simulink model "quadcopter"  (R2024a)
settings: Solver=ode45  StartTime=0.0  StopTime=100  FixedStep=0.0001  RelTol=1e-3
libraries: slpidlib x9
(part 1 of 2)
settings Model: Creator=ADMIN  LastModifiedBy=ADMIN

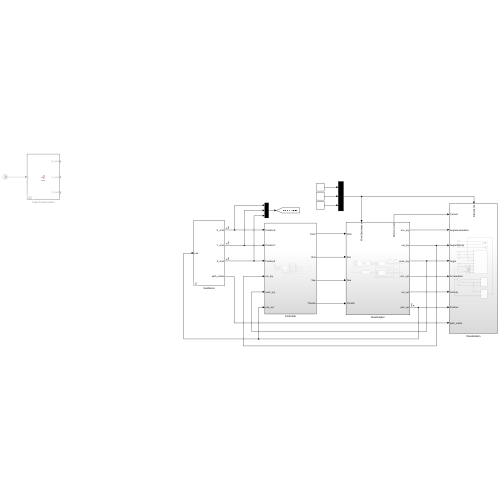
[thumbnail: Simulink's stored preview of the top-level diagram]
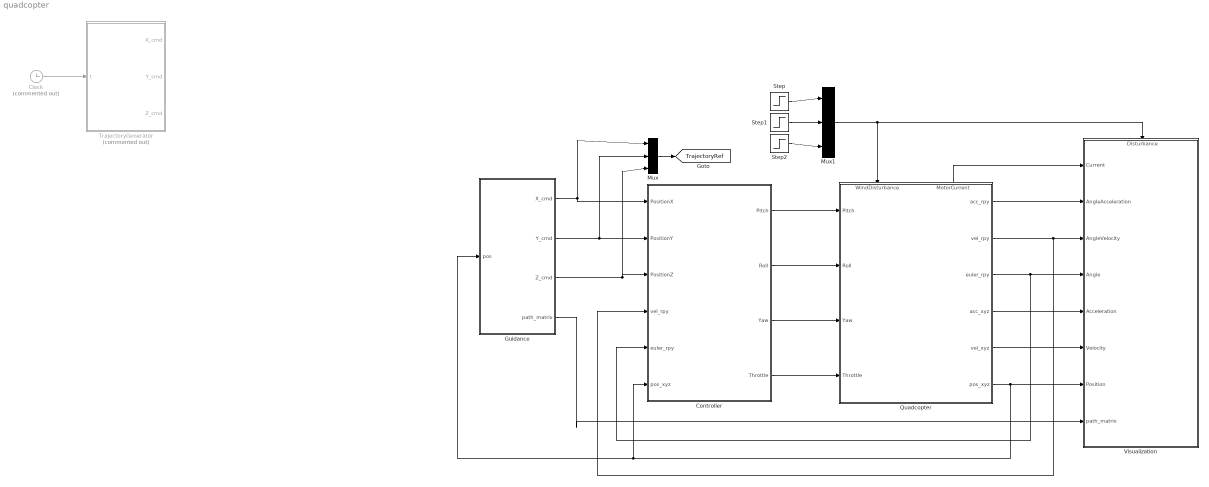
== system quadcopter ==
  Clock : Clock  Commented=on
  Controller : Subsystem
  Guidance : Subsystem  mask{trajectory_type=1}
      mask prompts: trajectory_type "helix: 1, figure-8: 2"
  Mux : Mux  Inputs=3
  Mux1 : Mux  Inputs=3
  Quadcopter : Subsystem
      settings: PortSchema="{\"entries\":[{\"content\":{\"sides\":[{\"content\":{\"connectorIds\":[\"In1\",\"In2\",\"In3\",\"In4\"]},\"type\":\"ConnectorPlacement.EquallySpacedRectSide\",\"uuid\":\"72979afb-3a13-47a6-b2df-41b5587480e1\"},{\"content\":{\"connectorIds\":[\"Out1\",\"Out2\",\"Out3\",\"Out4\",\"Out5\",\"Out6\"],\"side\":\"RIGHT\"},\"type\":\"ConnectorPlacement.EquallySpacedRectSide\",\"uuid\":\"ea12cd5a-a884-45c1-8d68-b4383d709346\"},{\"content\":{\"connectorIds\":[\"In5\",\"Out7\"],\"side\":\"TOP\"},\"type\":\"ConnectorPlacement.EquallySpacedRectSide\",\"uuid\":\"9fa1b2a5-ed05-4359-b2a5-dd09b0942958\"}]},\"type\":\"ConnectorPlacement.EquallySpacedConnector\",\"uuid\":\"94bc8a31-e0f4-4496-86b6-9264019e9c52\"}],\"packageUris\":[\"http://schema.mathworks.com/mf0/Connector/R2020b\"],\"version\":\"1.0\"}"
  Step : Step  Time=10  After=4  SampleTime=0
  Step1 : Step  Time=40  After=0  SampleTime=0
  Step2 : Step  Time=60  After=0  SampleTime=0
  TrajectoryGenerator : MATLAB Function  Commented=on  TreatAsAtomicUnit=on
  Visualization : Subsystem
      settings: PortSchema="{\"entries\":[{\"content\":{\"sides\":[{\"content\":{\"connectorIds\":[\"In1\",\"In2\",\"In3\",\"In4\",\"In5\",\"In6\",\"In7\",\"In8\"]},\"type\":\"ConnectorPlacement.EquallySpacedRectSide\",\"uuid\":\"3cb0b979-0d5f-4f09-adcd-90aa91650358\"},{\"content\":{\"side\":\"RIGHT\"},\"type\":\"ConnectorPlacement.EquallySpacedRectSide\",\"uuid\":\"d4f03e78-8acd-4062-a16e-5eca778df7bc\"},{\"content\":{\"connectorIds\":[\"In9\"],\"side\":\"TOP\"},\"type\":\"ConnectorPlacement.EquallySpacedRectSide\",\"uuid\":\"69a143a0-3c25-4fd4-9005-042b32bb0dbc\"}]},\"type\":\"ConnectorPlacement.EquallySpacedConnector\",\"uuid\":\"bd282390-c963-4ab6-a9ae-6b9e051d8e4c\"}],\"packageUris\":[\"http://schema.mathworks.com/mf0/Connector/R2020b\"],\"version\":\"1.0\"}"
  tag scope: TrajectoryRef=global
  wires:
  Quadcopter/6(pos_xyz) -> Guidance/1(pos), Controller/6(pos_xyz), Visualization/7(Position)
  Quadcopter/2(vel_rpy) -> Controller/4(vel_rpy), Visualization/3(AngleVelocity)
  Quadcopter/3(euler_rpy) -> Controller/5(euler_rpy), Visualization/4(Angle)
  Controller/1(Pitch) -> Quadcopter/1(Pitch)
  Controller/2(Roll) -> Quadcopter/2(Roll)
  Controller/3(Yaw) -> Quadcopter/3(Yaw)
  Controller/4(Throttle) -> Quadcopter/4(Throttle)
  Mux/1 -> [TrajectoryRef]
  Clock/1 -> TrajectoryGenerator/1(t)
  Guidance/3(Z_cmd) -> Controller/3(PositionZ), Mux/3
  Guidance/2(Y_cmd) -> Controller/2(PositionY), Mux/2
  Quadcopter/7(MotorCurrent) -> Visualization/1(Current)
  Quadcopter/1(acc_rpy) -> Visualization/2(AngleAcceleration)
  Guidance/4(path_matrix) -> Visualization/8(path_matrix)
  Quadcopter/4(acc_xyz) -> Visualization/5(Acceleration)
  Quadcopter/5(vel_xyz) -> Visualization/6(Velocity)
  Guidance/1(X_cmd) -> Mux/1, Controller/1(PositionX)
  Step/1 -> Mux1/1
  Step1/1 -> Mux1/2
  Step2/1 -> Mux1/3
  Mux1/1 -> Quadcopter/5(WindDisturbance), Visualization/9(Disturbance)

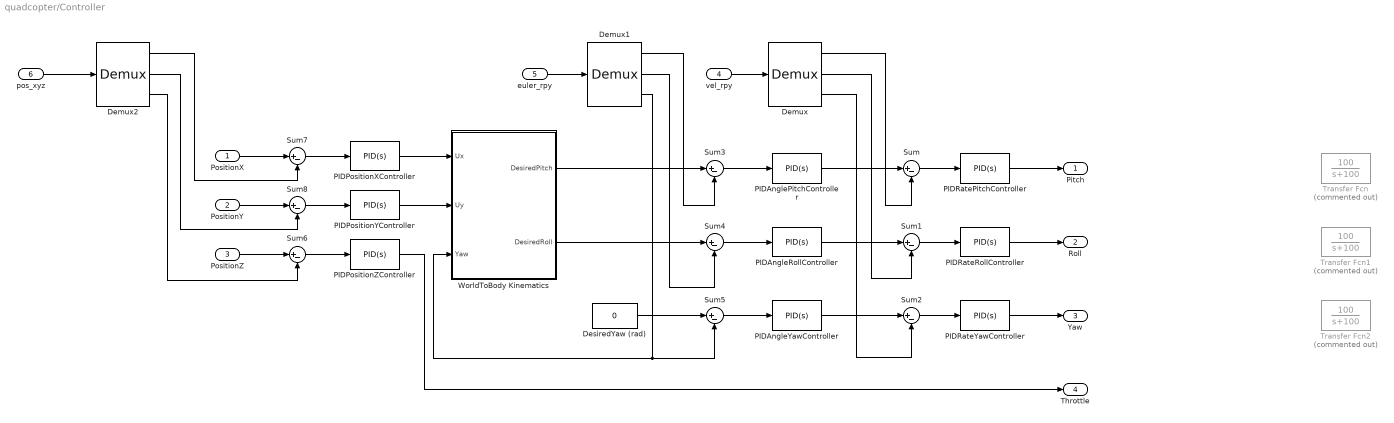
== system quadcopter/Controller ==
  PositionX : Inport
  PositionY : Inport  Port=2
  PositionZ : Inport  Port=3
  vel_rpy : Inport  Port=4
  euler_rpy : Inport  Port=5
  pos_xyz : Inport  Port=6
  Demux : Demux  Outputs=3
  Demux1 : Demux  Outputs=3
  Demux2 : Demux  Outputs=3
  DesiredYaw (rad) : Constant  Value=0
  PIDAnglePitchController : slpidlib/PID Controller  Controller=PID  Form=Parallel  TimeDomain=Continuous-time  UseExternalTs=off  SampleTime=-1  IntegratorMethod=Forward Euler  FilterMethod=Forward Euler  ControllerParametersSource=internal  P=10  I=5  UseKiTs=off  D=0  UseExternalDerivativeSource=off  N=100  UseFilter=on  TunerSelectOption=Transfer Function Based (PID Tuner App)  InitialConditionSource=internal  InitialConditionForIntegrator=0  InitialConditionForFilter=0  DifferentiatorICPrevScaledInput=0  ExternalReset=none  TrackingMode=off  Kt=1  LimitOutput=on  SatLimitsSource=internal  UpperSaturationLimit=50  LowerSaturationLimit=-50  LinearizeAsGain=on  AntiWindupMode=clamping  Kb=1  LimitIntegrator=off  UpperIntegratorSaturationLimit=inf  LowerIntegratorSaturationLimit=-inf  POutMin=[]  POutMax=[]  IOutMin=[]  IOutMax=[]  DOutMin=[]  DOutMax=[]  NOutMin=[]  NOutMax=[]  SumOutMin=[]  SumOutMax=[]  SaturationOutMin=[]  SaturationOutMax=[]  PParamMin=[]  PParamMax=[]  IParamMin=[]  IParamMax=[]  DParamMin=[]  DParamMax=[]  NParamMin=[]  NParamMax=[]  KbParamMin=[]  KbParamMax=[]  KtParamMin=[]  KtParamMax=[]  KbOutMin=[]  KbOutMax=[]  KtOutMin=[]  KtOutMax=[]  IntegratorOutMin=[]  IntegratorOutMax=[]  FilterOutMin=[]  FilterOutMax=[]  SumI1OutMin=[]  SumI1OutMax=[]  SumI2OutMin=[]  SumI2OutMax=[]  SumI3OutMin=[]  SumI3OutMax=[]  SumI4OutMin=[]  SumI4OutMax=[]  SumDOutMin=[]  SumDOutMax=[]  DifferentiatorOutMin=[]  DifferentiatorOutMax=[]  FilterDiffOutCoefMin=[]  FilterDiffOutCoefMax=[]  ReciprocalOutMin=[]  ReciprocalOutMax=[]  SumDenOutMin=[]  SumDenOutMax=[]  SumNumOutMin=[]  SumNumOutMax=[]  DivideOutMin=[]  DivideOutMax=[]  UdiffTsProdOutMin=[]  UdiffTsProdOutMax=[]  NTsProdOutMin=[]  NTsProdOutMax=[]  UintegralTsProdOutMin=[]  UintegralTsProdOutMax=[]  UngainTsProdOutMin=[]  UngainTsProdOutMax=[]  ClampingZeroOutDataTypeStr=Inherit: Inherit via back propagation  ClampingZeroOutMin=[]  ClampingZeroOutMax=[]  FilterDenConstantOutDataTypeStr=Inherit: Inherit via back propagation  FilterDenConstantOutMin=[]  FilterDenConstantOutMax=[]  PCopyOutDataTypeStr=Inherit: Inherit via back propagation  PCopyOutMin=[]  PCopyOutMax=[]  NCopyOutDataTypeStr=Inherit: Inherit via back propagation  NCopyOutMin=[]  NCopyOutMax=[]  IntegratorContinuousStateAttributes=''  IntegratorStateMustResolveToSignalObject=off  IntegratorRTWStateStorageClass=Auto  FilterContinuousStateAttributes=''  FilterStateMustResolveToSignalObject=off  FilterRTWStateStorageClass=Auto  ParallelPVariant=InternalParameters  IdealPVariant=Disabled  IVariant=InternalParameters  DVariant=InternalParameters  IntegratorVariant=Continuous  SatVariant=Enabled  AWVariant=ContClampingParallel  PCopyVariant=Disabled  TRVariant=Disabled  FdbkBlocksVariant=Forward  IdealPFdbkVariant=Disabled  SatFdbkVariant=Disabled  DerivativeFilterVariant=ContFilter  NVariant=InternalParameters  NCopyVariant=Disabled  FilterICVariant=InternalICsFilter  IntegratorICVariant=InternalICs  ExternalResetVariant=Disabled  TRSumVariant=Passthrough  SumFdbkVariant=Disabled  SumVariant=Sum_PID  TsampFilterVariant=InternalTs  TsampNgainVariant=Passthrough  TsampIntegralVariant=Disabled_SignalSpec  ExternalSaturationOutDataTypeStr=Inherit: Same as second input  DerivativeSourceVariant=ErrorSignal
  PIDAngleRollController : slpidlib/PID Controller  Controller=PID  Form=Parallel  TimeDomain=Continuous-time  UseExternalTs=off  SampleTime=-1  IntegratorMethod=Forward Euler  FilterMethod=Forward Euler  ControllerParametersSource=internal  P=10  I=5  UseKiTs=off  D=0  UseExternalDerivativeSource=off  N=100  UseFilter=on  TunerSelectOption=Transfer Function Based (PID Tuner App)  InitialConditionSource=internal  InitialConditionForIntegrator=0  InitialConditionForFilter=0  DifferentiatorICPrevScaledInput=0  ExternalReset=none  TrackingMode=off  Kt=1  LimitOutput=on  SatLimitsSource=internal  UpperSaturationLimit=50  LowerSaturationLimit=-50  LinearizeAsGain=on  AntiWindupMode=clamping  Kb=1  LimitIntegrator=off  UpperIntegratorSaturationLimit=inf  LowerIntegratorSaturationLimit=-inf  POutMin=[]  POutMax=[]  IOutMin=[]  IOutMax=[]  DOutMin=[]  DOutMax=[]  NOutMin=[]  NOutMax=[]  SumOutMin=[]  SumOutMax=[]  SaturationOutMin=[]  SaturationOutMax=[]  PParamMin=[]  PParamMax=[]  IParamMin=[]  IParamMax=[]  DParamMin=[]  DParamMax=[]  NParamMin=[]  NParamMax=[]  KbParamMin=[]  KbParamMax=[]  KtParamMin=[]  KtParamMax=[]  KbOutMin=[]  KbOutMax=[]  KtOutMin=[]  KtOutMax=[]  IntegratorOutMin=[]  IntegratorOutMax=[]  FilterOutMin=[]  FilterOutMax=[]  SumI1OutMin=[]  SumI1OutMax=[]  SumI2OutMin=[]  SumI2OutMax=[]  SumI3OutMin=[]  SumI3OutMax=[]  SumI4OutMin=[]  SumI4OutMax=[]  SumDOutMin=[]  SumDOutMax=[]  DifferentiatorOutMin=[]  DifferentiatorOutMax=[]  FilterDiffOutCoefMin=[]  FilterDiffOutCoefMax=[]  ReciprocalOutMin=[]  ReciprocalOutMax=[]  SumDenOutMin=[]  SumDenOutMax=[]  SumNumOutMin=[]  SumNumOutMax=[]  DivideOutMin=[]  DivideOutMax=[]  UdiffTsProdOutMin=[]  UdiffTsProdOutMax=[]  NTsProdOutMin=[]  NTsProdOutMax=[]  UintegralTsProdOutMin=[]  UintegralTsProdOutMax=[]  UngainTsProdOutMin=[]  UngainTsProdOutMax=[]  ClampingZeroOutDataTypeStr=Inherit: Inherit via back propagation  ClampingZeroOutMin=[]  ClampingZeroOutMax=[]  FilterDenConstantOutDataTypeStr=Inherit: Inherit via back propagation  FilterDenConstantOutMin=[]  FilterDenConstantOutMax=[]  PCopyOutDataTypeStr=Inherit: Inherit via back propagation  PCopyOutMin=[]  PCopyOutMax=[]  NCopyOutDataTypeStr=Inherit: Inherit via back propagation  NCopyOutMin=[]  NCopyOutMax=[]  IntegratorContinuousStateAttributes=''  IntegratorStateMustResolveToSignalObject=off  IntegratorRTWStateStorageClass=Auto  FilterContinuousStateAttributes=''  FilterStateMustResolveToSignalObject=off  FilterRTWStateStorageClass=Auto  ParallelPVariant=InternalParameters  IdealPVariant=Disabled  IVariant=InternalParameters  DVariant=InternalParameters  IntegratorVariant=Continuous  SatVariant=Enabled  AWVariant=ContClampingParallel  PCopyVariant=Disabled  TRVariant=Disabled  FdbkBlocksVariant=Forward  IdealPFdbkVariant=Disabled  SatFdbkVariant=Disabled  DerivativeFilterVariant=ContFilter  NVariant=InternalParameters  NCopyVariant=Disabled  FilterICVariant=InternalICsFilter  IntegratorICVariant=InternalICs  ExternalResetVariant=Disabled  TRSumVariant=Passthrough  SumFdbkVariant=Disabled  SumVariant=Sum_PID  TsampFilterVariant=InternalTs  TsampNgainVariant=Passthrough  TsampIntegralVariant=Disabled_SignalSpec  ExternalSaturationOutDataTypeStr=Inherit: Same as second input  DerivativeSourceVariant=ErrorSignal
  PIDAngleYawController : slpidlib/PID Controller  Controller=PID  Form=Parallel  TimeDomain=Continuous-time  UseExternalTs=off  SampleTime=-1  IntegratorMethod=Forward Euler  FilterMethod=Forward Euler  ControllerParametersSource=internal  P=10  I=0.5  UseKiTs=off  D=0  UseExternalDerivativeSource=off  N=100  UseFilter=on  TunerSelectOption=Transfer Function Based (PID Tuner App)  InitialConditionSource=internal  InitialConditionForIntegrator=0  InitialConditionForFilter=0  DifferentiatorICPrevScaledInput=0  ExternalReset=none  TrackingMode=off  Kt=1  LimitOutput=on  SatLimitsSource=internal  UpperSaturationLimit=50  LowerSaturationLimit=-50  LinearizeAsGain=on  AntiWindupMode=clamping  Kb=1  LimitIntegrator=off  UpperIntegratorSaturationLimit=inf  LowerIntegratorSaturationLimit=-inf  POutMin=[]  POutMax=[]  IOutMin=[]  IOutMax=[]  DOutMin=[]  DOutMax=[]  NOutMin=[]  NOutMax=[]  SumOutMin=[]  SumOutMax=[]  SaturationOutMin=[]  SaturationOutMax=[]  PParamMin=[]  PParamMax=[]  IParamMin=[]  IParamMax=[]  DParamMin=[]  DParamMax=[]  NParamMin=[]  NParamMax=[]  KbParamMin=[]  KbParamMax=[]  KtParamMin=[]  KtParamMax=[]  KbOutMin=[]  KbOutMax=[]  KtOutMin=[]  KtOutMax=[]  IntegratorOutMin=[]  IntegratorOutMax=[]  FilterOutMin=[]  FilterOutMax=[]  SumI1OutMin=[]  SumI1OutMax=[]  SumI2OutMin=[]  SumI2OutMax=[]  SumI3OutMin=[]  SumI3OutMax=[]  SumI4OutMin=[]  SumI4OutMax=[]  SumDOutMin=[]  SumDOutMax=[]  DifferentiatorOutMin=[]  DifferentiatorOutMax=[]  FilterDiffOutCoefMin=[]  FilterDiffOutCoefMax=[]  ReciprocalOutMin=[]  ReciprocalOutMax=[]  SumDenOutMin=[]  SumDenOutMax=[]  SumNumOutMin=[]  SumNumOutMax=[]  DivideOutMin=[]  DivideOutMax=[]  UdiffTsProdOutMin=[]  UdiffTsProdOutMax=[]  NTsProdOutMin=[]  NTsProdOutMax=[]  UintegralTsProdOutMin=[]  UintegralTsProdOutMax=[]  UngainTsProdOutMin=[]  UngainTsProdOutMax=[]  ClampingZeroOutDataTypeStr=Inherit: Inherit via back propagation  ClampingZeroOutMin=[]  ClampingZeroOutMax=[]  FilterDenConstantOutDataTypeStr=Inherit: Inherit via back propagation  FilterDenConstantOutMin=[]  FilterDenConstantOutMax=[]  PCopyOutDataTypeStr=Inherit: Inherit via back propagation  PCopyOutMin=[]  PCopyOutMax=[]  NCopyOutDataTypeStr=Inherit: Inherit via back propagation  NCopyOutMin=[]  NCopyOutMax=[]  IntegratorContinuousStateAttributes=''  IntegratorStateMustResolveToSignalObject=off  IntegratorRTWStateStorageClass=Auto  FilterContinuousStateAttributes=''  FilterStateMustResolveToSignalObject=off  FilterRTWStateStorageClass=Auto  ParallelPVariant=InternalParameters  IdealPVariant=Disabled  IVariant=InternalParameters  DVariant=InternalParameters  IntegratorVariant=Continuous  SatVariant=Enabled  AWVariant=ContClampingParallel  PCopyVariant=Disabled  TRVariant=Disabled  FdbkBlocksVariant=Forward  IdealPFdbkVariant=Disabled  SatFdbkVariant=Disabled  DerivativeFilterVariant=ContFilter  NVariant=InternalParameters  NCopyVariant=Disabled  FilterICVariant=InternalICsFilter  IntegratorICVariant=InternalICs  ExternalResetVariant=Disabled  TRSumVariant=Passthrough  SumFdbkVariant=Disabled  SumVariant=Sum_PID  TsampFilterVariant=InternalTs  TsampNgainVariant=Passthrough  TsampIntegralVariant=Disabled_SignalSpec  ExternalSaturationOutDataTypeStr=Inherit: Same as second input  DerivativeSourceVariant=ErrorSignal
  PIDPositionXController : slpidlib/PID Controller  Controller=PID  Form=Parallel  TimeDomain=Continuous-time  UseExternalTs=off  SampleTime=-1  IntegratorMethod=Forward Euler  FilterMethod=Forward Euler  ControllerParametersSource=internal  P=0.05  I=0  UseKiTs=off  D=0.15  UseExternalDerivativeSource=off  N=100  UseFilter=on  TunerSelectOption=Transfer Function Based (PID Tuner App)  InitialConditionSource=internal  InitialConditionForIntegrator=0  InitialConditionForFilter=0  DifferentiatorICPrevScaledInput=0  ExternalReset=none  TrackingMode=off  Kt=1  LimitOutput=on  SatLimitsSource=internal  UpperSaturationLimit=0.35  LowerSaturationLimit=-0.35  LinearizeAsGain=on  AntiWindupMode=clamping  Kb=1  LimitIntegrator=off  UpperIntegratorSaturationLimit=inf  LowerIntegratorSaturationLimit=-inf  POutMin=[]  POutMax=[]  IOutMin=[]  IOutMax=[]  DOutMin=[]  DOutMax=[]  NOutMin=[]  NOutMax=[]  SumOutMin=[]  SumOutMax=[]  SaturationOutMin=[]  SaturationOutMax=[]  PParamMin=[]  PParamMax=[]  IParamMin=[]  IParamMax=[]  DParamMin=[]  DParamMax=[]  NParamMin=[]  NParamMax=[]  KbParamMin=[]  KbParamMax=[]  KtParamMin=[]  KtParamMax=[]  KbOutMin=[]  KbOutMax=[]  KtOutMin=[]  KtOutMax=[]  IntegratorOutMin=[]  IntegratorOutMax=[]  FilterOutMin=[]  FilterOutMax=[]  SumI1OutMin=[]  SumI1OutMax=[]  SumI2OutMin=[]  SumI2OutMax=[]  SumI3OutMin=[]  SumI3OutMax=[]  SumI4OutMin=[]  SumI4OutMax=[]  SumDOutMin=[]  SumDOutMax=[]  DifferentiatorOutMin=[]  DifferentiatorOutMax=[]  FilterDiffOutCoefMin=[]  FilterDiffOutCoefMax=[]  ReciprocalOutMin=[]  ReciprocalOutMax=[]  SumDenOutMin=[]  SumDenOutMax=[]  SumNumOutMin=[]  SumNumOutMax=[]  DivideOutMin=[]  DivideOutMax=[]  UdiffTsProdOutMin=[]  UdiffTsProdOutMax=[]  NTsProdOutMin=[]  NTsProdOutMax=[]  UintegralTsProdOutMin=[]  UintegralTsProdOutMax=[]  UngainTsProdOutMin=[]  UngainTsProdOutMax=[]  ClampingZeroOutDataTypeStr=Inherit: Inherit via back propagation  ClampingZeroOutMin=[]  ClampingZeroOutMax=[]  FilterDenConstantOutDataTypeStr=Inherit: Inherit via back propagation  FilterDenConstantOutMin=[]  FilterDenConstantOutMax=[]  PCopyOutDataTypeStr=Inherit: Inherit via back propagation  PCopyOutMin=[]  PCopyOutMax=[]  NCopyOutDataTypeStr=Inherit: Inherit via back propagation  NCopyOutMin=[]  NCopyOutMax=[]  IntegratorContinuousStateAttributes=''  IntegratorStateMustResolveToSignalObject=off  IntegratorRTWStateStorageClass=Auto  FilterContinuousStateAttributes=''  FilterStateMustResolveToSignalObject=off  FilterRTWStateStorageClass=Auto  ParallelPVariant=InternalParameters  IdealPVariant=Disabled  IVariant=InternalParameters  DVariant=InternalParameters  IntegratorVariant=Continuous  SatVariant=Enabled  AWVariant=ContClampingParallel  PCopyVariant=Disabled  TRVariant=Disabled  FdbkBlocksVariant=Forward  IdealPFdbkVariant=Disabled  SatFdbkVariant=Disabled  DerivativeFilterVariant=ContFilter  NVariant=InternalParameters  NCopyVariant=Disabled  FilterICVariant=InternalICsFilter  IntegratorICVariant=InternalICs  ExternalResetVariant=Disabled  TRSumVariant=Passthrough  SumFdbkVariant=Disabled  SumVariant=Sum_PID  TsampFilterVariant=InternalTs  TsampNgainVariant=Passthrough  TsampIntegralVariant=Disabled_SignalSpec  ExternalSaturationOutDataTypeStr=Inherit: Same as second input  DerivativeSourceVariant=ErrorSignal
  PIDPositionYController : slpidlib/PID Controller  Controller=PID  Form=Parallel  TimeDomain=Continuous-time  UseExternalTs=off  SampleTime=-1  IntegratorMethod=Forward Euler  FilterMethod=Forward Euler  ControllerParametersSource=internal  P=0.05  I=0  UseKiTs=off  D=0.15  UseExternalDerivativeSource=off  N=100  UseFilter=on  TunerSelectOption=Transfer Function Based (PID Tuner App)  InitialConditionSource=internal  InitialConditionForIntegrator=0  InitialConditionForFilter=0  DifferentiatorICPrevScaledInput=0  ExternalReset=none  TrackingMode=off  Kt=1  LimitOutput=on  SatLimitsSource=internal  UpperSaturationLimit=0.35  LowerSaturationLimit=-0.35  LinearizeAsGain=on  AntiWindupMode=clamping  Kb=1  LimitIntegrator=off  UpperIntegratorSaturationLimit=inf  LowerIntegratorSaturationLimit=-inf  POutMin=[]  POutMax=[]  IOutMin=[]  IOutMax=[]  DOutMin=[]  DOutMax=[]  NOutMin=[]  NOutMax=[]  SumOutMin=[]  SumOutMax=[]  SaturationOutMin=[]  SaturationOutMax=[]  PParamMin=[]  PParamMax=[]  IParamMin=[]  IParamMax=[]  DParamMin=[]  DParamMax=[]  NParamMin=[]  NParamMax=[]  KbParamMin=[]  KbParamMax=[]  KtParamMin=[]  KtParamMax=[]  KbOutMin=[]  KbOutMax=[]  KtOutMin=[]  KtOutMax=[]  IntegratorOutMin=[]  IntegratorOutMax=[]  FilterOutMin=[]  FilterOutMax=[]  SumI1OutMin=[]  SumI1OutMax=[]  SumI2OutMin=[]  SumI2OutMax=[]  SumI3OutMin=[]  SumI3OutMax=[]  SumI4OutMin=[]  SumI4OutMax=[]  SumDOutMin=[]  SumDOutMax=[]  DifferentiatorOutMin=[]  DifferentiatorOutMax=[]  FilterDiffOutCoefMin=[]  FilterDiffOutCoefMax=[]  ReciprocalOutMin=[]  ReciprocalOutMax=[]  SumDenOutMin=[]  SumDenOutMax=[]  SumNumOutMin=[]  SumNumOutMax=[]  DivideOutMin=[]  DivideOutMax=[]  UdiffTsProdOutMin=[]  UdiffTsProdOutMax=[]  NTsProdOutMin=[]  NTsProdOutMax=[]  UintegralTsProdOutMin=[]  UintegralTsProdOutMax=[]  UngainTsProdOutMin=[]  UngainTsProdOutMax=[]  ClampingZeroOutDataTypeStr=Inherit: Inherit via back propagation  ClampingZeroOutMin=[]  ClampingZeroOutMax=[]  FilterDenConstantOutDataTypeStr=Inherit: Inherit via back propagation  FilterDenConstantOutMin=[]  FilterDenConstantOutMax=[]  PCopyOutDataTypeStr=Inherit: Inherit via back propagation  PCopyOutMin=[]  PCopyOutMax=[]  NCopyOutDataTypeStr=Inherit: Inherit via back propagation  NCopyOutMin=[]  NCopyOutMax=[]  IntegratorContinuousStateAttributes=''  IntegratorStateMustResolveToSignalObject=off  IntegratorRTWStateStorageClass=Auto  FilterContinuousStateAttributes=''  FilterStateMustResolveToSignalObject=off  FilterRTWStateStorageClass=Auto  ParallelPVariant=InternalParameters  IdealPVariant=Disabled  IVariant=InternalParameters  DVariant=InternalParameters  IntegratorVariant=Continuous  SatVariant=Enabled  AWVariant=ContClampingParallel  PCopyVariant=Disabled  TRVariant=Disabled  FdbkBlocksVariant=Forward  IdealPFdbkVariant=Disabled  SatFdbkVariant=Disabled  DerivativeFilterVariant=ContFilter  NVariant=InternalParameters  NCopyVariant=Disabled  FilterICVariant=InternalICsFilter  IntegratorICVariant=InternalICs  ExternalResetVariant=Disabled  TRSumVariant=Passthrough  SumFdbkVariant=Disabled  SumVariant=Sum_PID  TsampFilterVariant=InternalTs  TsampNgainVariant=Passthrough  TsampIntegralVariant=Disabled_SignalSpec  ExternalSaturationOutDataTypeStr=Inherit: Same as second input  DerivativeSourceVariant=ErrorSignal
  PIDPositionZController : slpidlib/PID Controller  Controller=PID  Form=Parallel  TimeDomain=Continuous-time  UseExternalTs=off  SampleTime=-1  IntegratorMethod=Forward Euler  FilterMethod=Forward Euler  ControllerParametersSource=internal  P=15  I=5  UseKiTs=off  D=10  UseExternalDerivativeSource=off  N=100  UseFilter=on  TunerSelectOption=Transfer Function Based (PID Tuner App)  InitialConditionSource=internal  InitialConditionForIntegrator=0  InitialConditionForFilter=0  DifferentiatorICPrevScaledInput=0  ExternalReset=none  TrackingMode=off  Kt=1  LimitOutput=on  SatLimitsSource=internal  UpperSaturationLimit=100  LowerSaturationLimit=0  LinearizeAsGain=on  AntiWindupMode=clamping  Kb=1  LimitIntegrator=off  UpperIntegratorSaturationLimit=inf  LowerIntegratorSaturationLimit=-inf  POutMin=[]  POutMax=[]  IOutMin=[]  IOutMax=[]  DOutMin=[]  DOutMax=[]  NOutMin=[]  NOutMax=[]  SumOutMin=[]  SumOutMax=[]  SaturationOutMin=[]  SaturationOutMax=[]  PParamMin=[]  PParamMax=[]  IParamMin=[]  IParamMax=[]  DParamMin=[]  DParamMax=[]  NParamMin=[]  NParamMax=[]  KbParamMin=[]  KbParamMax=[]  KtParamMin=[]  KtParamMax=[]  KbOutMin=[]  KbOutMax=[]  KtOutMin=[]  KtOutMax=[]  IntegratorOutMin=[]  IntegratorOutMax=[]  FilterOutMin=[]  FilterOutMax=[]  SumI1OutMin=[]  SumI1OutMax=[]  SumI2OutMin=[]  SumI2OutMax=[]  SumI3OutMin=[]  SumI3OutMax=[]  SumI4OutMin=[]  SumI4OutMax=[]  SumDOutMin=[]  SumDOutMax=[]  DifferentiatorOutMin=[]  DifferentiatorOutMax=[]  FilterDiffOutCoefMin=[]  FilterDiffOutCoefMax=[]  ReciprocalOutMin=[]  ReciprocalOutMax=[]  SumDenOutMin=[]  SumDenOutMax=[]  SumNumOutMin=[]  SumNumOutMax=[]  DivideOutMin=[]  DivideOutMax=[]  UdiffTsProdOutMin=[]  UdiffTsProdOutMax=[]  NTsProdOutMin=[]  NTsProdOutMax=[]  UintegralTsProdOutMin=[]  UintegralTsProdOutMax=[]  UngainTsProdOutMin=[]  UngainTsProdOutMax=[]  ClampingZeroOutDataTypeStr=Inherit: Inherit via back propagation  ClampingZeroOutMin=[]  ClampingZeroOutMax=[]  FilterDenConstantOutDataTypeStr=Inherit: Inherit via back propagation  FilterDenConstantOutMin=[]  FilterDenConstantOutMax=[]  PCopyOutDataTypeStr=Inherit: Inherit via back propagation  PCopyOutMin=[]  PCopyOutMax=[]  NCopyOutDataTypeStr=Inherit: Inherit via back propagation  NCopyOutMin=[]  NCopyOutMax=[]  IntegratorContinuousStateAttributes=''  IntegratorStateMustResolveToSignalObject=off  IntegratorRTWStateStorageClass=Auto  FilterContinuousStateAttributes=''  FilterStateMustResolveToSignalObject=off  FilterRTWStateStorageClass=Auto  ParallelPVariant=InternalParameters  IdealPVariant=Disabled  IVariant=InternalParameters  DVariant=InternalParameters  IntegratorVariant=Continuous  SatVariant=Enabled  AWVariant=ContClampingParallel  PCopyVariant=Disabled  TRVariant=Disabled  FdbkBlocksVariant=Forward  IdealPFdbkVariant=Disabled  SatFdbkVariant=Disabled  DerivativeFilterVariant=ContFilter  NVariant=InternalParameters  NCopyVariant=Disabled  FilterICVariant=InternalICsFilter  IntegratorICVariant=InternalICs  ExternalResetVariant=Disabled  TRSumVariant=Passthrough  SumFdbkVariant=Disabled  SumVariant=Sum_PID  TsampFilterVariant=InternalTs  TsampNgainVariant=Passthrough  TsampIntegralVariant=Disabled_SignalSpec  ExternalSaturationOutDataTypeStr=Inherit: Same as second input  DerivativeSourceVariant=ErrorSignal
  PIDRatePitchController : slpidlib/PID Controller  Controller=PID  Form=Parallel  TimeDomain=Continuous-time  UseExternalTs=off  SampleTime=-1  IntegratorMethod=Forward Euler  FilterMethod=Forward Euler  ControllerParametersSource=internal  P=10  I=5  UseKiTs=off  D=0  UseExternalDerivativeSource=off  N=100  UseFilter=on  TunerSelectOption=Transfer Function Based (PID Tuner App)  InitialConditionSource=internal  InitialConditionForIntegrator=0  InitialConditionForFilter=0  DifferentiatorICPrevScaledInput=0  ExternalReset=none  TrackingMode=off  Kt=1  LimitOutput=on  SatLimitsSource=internal  UpperSaturationLimit=100  LowerSaturationLimit=-100  LinearizeAsGain=on  AntiWindupMode=clamping  Kb=1  LimitIntegrator=off  UpperIntegratorSaturationLimit=inf  LowerIntegratorSaturationLimit=-inf  POutMin=[]  POutMax=[]  IOutMin=[]  IOutMax=[]  DOutMin=[]  DOutMax=[]  NOutMin=[]  NOutMax=[]  SumOutMin=[]  SumOutMax=[]  SaturationOutMin=[]  SaturationOutMax=[]  PParamMin=[]  PParamMax=[]  IParamMin=[]  IParamMax=[]  DParamMin=[]  DParamMax=[]  NParamMin=[]  NParamMax=[]  KbParamMin=[]  KbParamMax=[]  KtParamMin=[]  KtParamMax=[]  KbOutMin=[]  KbOutMax=[]  KtOutMin=[]  KtOutMax=[]  IntegratorOutMin=[]  IntegratorOutMax=[]  FilterOutMin=[]  FilterOutMax=[]  SumI1OutMin=[]  SumI1OutMax=[]  SumI2OutMin=[]  SumI2OutMax=[]  SumI3OutMin=[]  SumI3OutMax=[]  SumI4OutMin=[]  SumI4OutMax=[]  SumDOutMin=[]  SumDOutMax=[]  DifferentiatorOutMin=[]  DifferentiatorOutMax=[]  FilterDiffOutCoefMin=[]  FilterDiffOutCoefMax=[]  ReciprocalOutMin=[]  ReciprocalOutMax=[]  SumDenOutMin=[]  SumDenOutMax=[]  SumNumOutMin=[]  SumNumOutMax=[]  DivideOutMin=[]  DivideOutMax=[]  UdiffTsProdOutMin=[]  UdiffTsProdOutMax=[]  NTsProdOutMin=[]  NTsProdOutMax=[]  UintegralTsProdOutMin=[]  UintegralTsProdOutMax=[]  UngainTsProdOutMin=[]  UngainTsProdOutMax=[]  ClampingZeroOutDataTypeStr=Inherit: Inherit via back propagation  ClampingZeroOutMin=[]  ClampingZeroOutMax=[]  FilterDenConstantOutDataTypeStr=Inherit: Inherit via back propagation  FilterDenConstantOutMin=[]  FilterDenConstantOutMax=[]  PCopyOutDataTypeStr=Inherit: Inherit via back propagation  PCopyOutMin=[]  PCopyOutMax=[]  NCopyOutDataTypeStr=Inherit: Inherit via back propagation  NCopyOutMin=[]  NCopyOutMax=[]  IntegratorContinuousStateAttributes=''  IntegratorStateMustResolveToSignalObject=off  IntegratorRTWStateStorageClass=Auto  FilterContinuousStateAttributes=''  FilterStateMustResolveToSignalObject=off  FilterRTWStateStorageClass=Auto  ParallelPVariant=InternalParameters  IdealPVariant=Disabled  IVariant=InternalParameters  DVariant=InternalParameters  IntegratorVariant=Continuous  SatVariant=Enabled  AWVariant=ContClampingParallel  PCopyVariant=Disabled  TRVariant=Disabled  FdbkBlocksVariant=Forward  IdealPFdbkVariant=Disabled  SatFdbkVariant=Disabled  DerivativeFilterVariant=ContFilter  NVariant=InternalParameters  NCopyVariant=Disabled  FilterICVariant=InternalICsFilter  IntegratorICVariant=InternalICs  ExternalResetVariant=Disabled  TRSumVariant=Passthrough  SumFdbkVariant=Disabled  SumVariant=Sum_PID  TsampFilterVariant=InternalTs  TsampNgainVariant=Passthrough  TsampIntegralVariant=Disabled_SignalSpec  ExternalSaturationOutDataTypeStr=Inherit: Same as second input  DerivativeSourceVariant=ErrorSignal
  PIDRateRollController : slpidlib/PID Controller  Controller=PID  Form=Parallel  TimeDomain=Continuous-time  UseExternalTs=off  SampleTime=-1  IntegratorMethod=Forward Euler  FilterMethod=Forward Euler  ControllerParametersSource=internal  P=20  I=5  UseKiTs=off  D=0  UseExternalDerivativeSource=off  N=100  UseFilter=on  TunerSelectOption=Transfer Function Based (PID Tuner App)  InitialConditionSource=internal  InitialConditionForIntegrator=0  InitialConditionForFilter=0  DifferentiatorICPrevScaledInput=0  ExternalReset=none  TrackingMode=off  Kt=1  LimitOutput=on  SatLimitsSource=internal  UpperSaturationLimit=100  LowerSaturationLimit=-100  LinearizeAsGain=on  AntiWindupMode=clamping  Kb=1  LimitIntegrator=off  UpperIntegratorSaturationLimit=inf  LowerIntegratorSaturationLimit=-inf  POutMin=[]  POutMax=[]  IOutMin=[]  IOutMax=[]  DOutMin=[]  DOutMax=[]  NOutMin=[]  NOutMax=[]  SumOutMin=[]  SumOutMax=[]  SaturationOutMin=[]  SaturationOutMax=[]  PParamMin=[]  PParamMax=[]  IParamMin=[]  IParamMax=[]  DParamMin=[]  DParamMax=[]  NParamMin=[]  NParamMax=[]  KbParamMin=[]  KbParamMax=[]  KtParamMin=[]  KtParamMax=[]  KbOutMin=[]  KbOutMax=[]  KtOutMin=[]  KtOutMax=[]  IntegratorOutMin=[]  IntegratorOutMax=[]  FilterOutMin=[]  FilterOutMax=[]  SumI1OutMin=[]  SumI1OutMax=[]  SumI2OutMin=[]  SumI2OutMax=[]  SumI3OutMin=[]  SumI3OutMax=[]  SumI4OutMin=[]  SumI4OutMax=[]  SumDOutMin=[]  SumDOutMax=[]  DifferentiatorOutMin=[]  DifferentiatorOutMax=[]  FilterDiffOutCoefMin=[]  FilterDiffOutCoefMax=[]  ReciprocalOutMin=[]  ReciprocalOutMax=[]  SumDenOutMin=[]  SumDenOutMax=[]  SumNumOutMin=[]  SumNumOutMax=[]  DivideOutMin=[]  DivideOutMax=[]  UdiffTsProdOutMin=[]  UdiffTsProdOutMax=[]  NTsProdOutMin=[]  NTsProdOutMax=[]  UintegralTsProdOutMin=[]  UintegralTsProdOutMax=[]  UngainTsProdOutMin=[]  UngainTsProdOutMax=[]  ClampingZeroOutDataTypeStr=Inherit: Inherit via back propagation  ClampingZeroOutMin=[]  ClampingZeroOutMax=[]  FilterDenConstantOutDataTypeStr=Inherit: Inherit via back propagation  FilterDenConstantOutMin=[]  FilterDenConstantOutMax=[]  PCopyOutDataTypeStr=Inherit: Inherit via back propagation  PCopyOutMin=[]  PCopyOutMax=[]  NCopyOutDataTypeStr=Inherit: Inherit via back propagation  NCopyOutMin=[]  NCopyOutMax=[]  IntegratorContinuousStateAttributes=''  IntegratorStateMustResolveToSignalObject=off  IntegratorRTWStateStorageClass=Auto  FilterContinuousStateAttributes=''  FilterStateMustResolveToSignalObject=off  FilterRTWStateStorageClass=Auto  ParallelPVariant=InternalParameters  IdealPVariant=Disabled  IVariant=InternalParameters  DVariant=InternalParameters  IntegratorVariant=Continuous  SatVariant=Enabled  AWVariant=ContClampingParallel  PCopyVariant=Disabled  TRVariant=Disabled  FdbkBlocksVariant=Forward  IdealPFdbkVariant=Disabled  SatFdbkVariant=Disabled  DerivativeFilterVariant=ContFilter  NVariant=InternalParameters  NCopyVariant=Disabled  FilterICVariant=InternalICsFilter  IntegratorICVariant=InternalICs  ExternalResetVariant=Disabled  TRSumVariant=Passthrough  SumFdbkVariant=Disabled  SumVariant=Sum_PID  TsampFilterVariant=InternalTs  TsampNgainVariant=Passthrough  TsampIntegralVariant=Disabled_SignalSpec  ExternalSaturationOutDataTypeStr=Inherit: Same as second input  DerivativeSourceVariant=ErrorSignal
  PIDRateYawController : slpidlib/PID Controller  Controller=PID  Form=Parallel  TimeDomain=Continuous-time  UseExternalTs=off  SampleTime=-1  IntegratorMethod=Forward Euler  FilterMethod=Forward Euler  ControllerParametersSource=internal  P=10  I=0.5  UseKiTs=off  D=0  UseExternalDerivativeSource=off  N=100  UseFilter=on  TunerSelectOption=Transfer Function Based (PID Tuner App)  InitialConditionSource=internal  InitialConditionForIntegrator=0  InitialConditionForFilter=0  DifferentiatorICPrevScaledInput=0  ExternalReset=none  TrackingMode=off  Kt=1  LimitOutput=on  SatLimitsSource=internal  UpperSaturationLimit=100  LowerSaturationLimit=-100  LinearizeAsGain=on  AntiWindupMode=clamping  Kb=1  LimitIntegrator=off  UpperIntegratorSaturationLimit=inf  LowerIntegratorSaturationLimit=-inf  POutMin=[]  POutMax=[]  IOutMin=[]  IOutMax=[]  DOutMin=[]  DOutMax=[]  NOutMin=[]  NOutMax=[]  SumOutMin=[]  SumOutMax=[]  SaturationOutMin=[]  SaturationOutMax=[]  PParamMin=[]  PParamMax=[]  IParamMin=[]  IParamMax=[]  DParamMin=[]  DParamMax=[]  NParamMin=[]  NParamMax=[]  KbParamMin=[]  KbParamMax=[]  KtParamMin=[]  KtParamMax=[]  KbOutMin=[]  KbOutMax=[]  KtOutMin=[]  KtOutMax=[]  IntegratorOutMin=[]  IntegratorOutMax=[]  FilterOutMin=[]  FilterOutMax=[]  SumI1OutMin=[]  SumI1OutMax=[]  SumI2OutMin=[]  SumI2OutMax=[]  SumI3OutMin=[]  SumI3OutMax=[]  SumI4OutMin=[]  SumI4OutMax=[]  SumDOutMin=[]  SumDOutMax=[]  DifferentiatorOutMin=[]  DifferentiatorOutMax=[]  FilterDiffOutCoefMin=[]  FilterDiffOutCoefMax=[]  ReciprocalOutMin=[]  ReciprocalOutMax=[]  SumDenOutMin=[]  SumDenOutMax=[]  SumNumOutMin=[]  SumNumOutMax=[]  DivideOutMin=[]  DivideOutMax=[]  UdiffTsProdOutMin=[]  UdiffTsProdOutMax=[]  NTsProdOutMin=[]  NTsProdOutMax=[]  UintegralTsProdOutMin=[]  UintegralTsProdOutMax=[]  UngainTsProdOutMin=[]  UngainTsProdOutMax=[]  ClampingZeroOutDataTypeStr=Inherit: Inherit via back propagation  ClampingZeroOutMin=[]  ClampingZeroOutMax=[]  FilterDenConstantOutDataTypeStr=Inherit: Inherit via back propagation  FilterDenConstantOutMin=[]  FilterDenConstantOutMax=[]  PCopyOutDataTypeStr=Inherit: Inherit via back propagation  PCopyOutMin=[]  PCopyOutMax=[]  NCopyOutDataTypeStr=Inherit: Inherit via back propagation  NCopyOutMin=[]  NCopyOutMax=[]  IntegratorContinuousStateAttributes=''  IntegratorStateMustResolveToSignalObject=off  IntegratorRTWStateStorageClass=Auto  FilterContinuousStateAttributes=''  FilterStateMustResolveToSignalObject=off  FilterRTWStateStorageClass=Auto  ParallelPVariant=InternalParameters  IdealPVariant=Disabled  IVariant=InternalParameters  DVariant=InternalParameters  IntegratorVariant=Continuous  SatVariant=Enabled  AWVariant=ContClampingParallel  PCopyVariant=Disabled  TRVariant=Disabled  FdbkBlocksVariant=Forward  IdealPFdbkVariant=Disabled  SatFdbkVariant=Disabled  DerivativeFilterVariant=ContFilter  NVariant=InternalParameters  NCopyVariant=Disabled  FilterICVariant=InternalICsFilter  IntegratorICVariant=InternalICs  ExternalResetVariant=Disabled  TRSumVariant=Passthrough  SumFdbkVariant=Disabled  SumVariant=Sum_PID  TsampFilterVariant=InternalTs  TsampNgainVariant=Passthrough  TsampIntegralVariant=Disabled_SignalSpec  ExternalSaturationOutDataTypeStr=Inherit: Same as second input  DerivativeSourceVariant=ErrorSignal
  Sum{,1..8} (9 alike) : Sum  Inputs=|+-
  Transfer Fcn : TransferFcn  Commented=on  Numerator=[100]  Denominator=[1 100]
  Transfer Fcn1 : TransferFcn  Commented=on  Numerator=[100]  Denominator=[1 100]
  Transfer Fcn2 : TransferFcn  Commented=on  Numerator=[100]  Denominator=[1 100]
  WorldToBody Kinematics : MATLAB Function  TreatAsAtomicUnit=on
  Pitch : Outport
  Roll : Outport  Port=2
  Yaw : Outport  Port=3
  Throttle : Outport  Port=4
  wires:
  DesiredYaw (rad)/1 -> Sum5/1
  Demux/2 -> Sum1/2
  Sum/1 -> PIDRatePitchController/1
  PIDPositionZController/1 -> Throttle/1
  Demux1/1 -> Sum3/2
  Sum5/1 -> PIDAngleYawController/1
  Demux1/2 -> Sum4/2
  Sum3/1 -> PIDAnglePitchController/1
  Sum4/1 -> PIDAngleRollController/1
  Demux/1 -> Sum/2
  Demux2/3 -> Sum6/2
  Sum2/1 -> PIDRateYawController/1
  Sum6/1 -> PIDPositionZController/1
  Demux2/1 -> Sum7/2
  Sum8/1 -> PIDPositionYController/1
  Sum7/1 -> PIDPositionXController/1
  vel_rpy/1 -> Demux/1
  Sum1/1 -> PIDRateRollController/1
  Demux1/3 -> Sum5/2, WorldToBody Kinematics/3(Yaw)
  PIDPositionYController/1 -> WorldToBody Kinematics/2(Uy)
  WorldToBody Kinematics/1(DesiredPitch) -> Sum3/1
  Demux/3 -> Sum2/2
  WorldToBody Kinematics/2(DesiredRoll) -> Sum4/1
  PIDPositionXController/1 -> WorldToBody Kinematics/1(Ux)
  euler_rpy/1 -> Demux1/1
  Demux2/2 -> Sum8/2
  pos_xyz/1 -> Demux2/1
  PositionX/1 -> Sum7/1
  PositionY/1 -> Sum8/1
  PositionZ/1 -> Sum6/1
  PIDRatePitchController/1 -> Pitch/1
  PIDRateRollController/1 -> Roll/1
  PIDRateYawController/1 -> Yaw/1
  PIDAnglePitchController/1 -> Sum/1
  PIDAngleRollController/1 -> Sum1/1
  PIDAngleYawController/1 -> Sum2/1

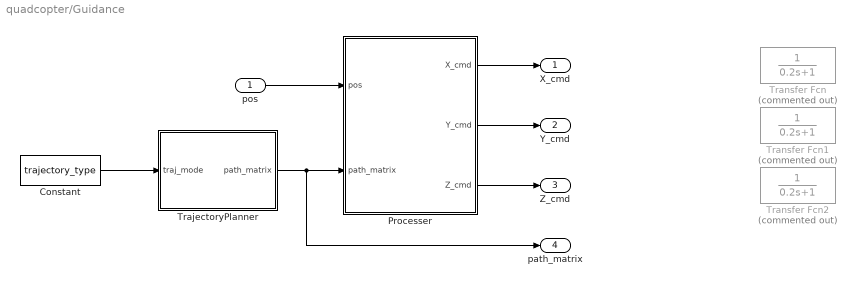
== system quadcopter/Guidance ==
  pos : Inport
  Constant : Constant  Value=trajectory_type
  Processer : MATLAB Function  TreatAsAtomicUnit=on
  TrajectoryPlanner : MATLAB Function  TreatAsAtomicUnit=on
  Transfer Fcn : TransferFcn  Commented=on  Denominator=[0.2 1]
  Transfer Fcn1 : TransferFcn  Commented=on  Denominator=[0.2 1]
  Transfer Fcn2 : TransferFcn  Commented=on  Denominator=[0.2 1]
  X_cmd : Outport
  Y_cmd : Outport  Port=2
  Z_cmd : Outport  Port=3
  path_matrix : Outport  Port=4
  wires:
  pos/1 -> Processer/1(pos)
  TrajectoryPlanner/1(path_matrix) -> path_matrix/1, Processer/2(path_matrix)
  Constant/1 -> TrajectoryPlanner/1(traj_mode)
  Processer/1(X_cmd) -> X_cmd/1
  Processer/2(Y_cmd) -> Y_cmd/1
  Processer/3(Z_cmd) -> Z_cmd/1

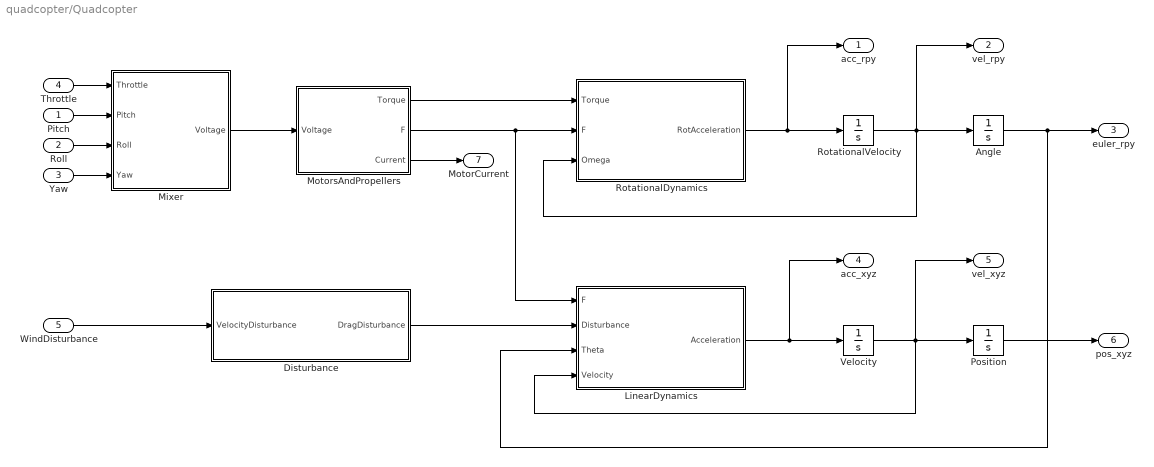
== system quadcopter/Quadcopter ==
  Pitch : Inport
  Roll : Inport  Port=2
  Yaw : Inport  Port=3
  Throttle : Inport  Port=4
  WindDisturbance : Inport  Port=5
  Angle : Integrator
  Disturbance : MATLAB Function  TreatAsAtomicUnit=on
  LinearDynamics : MATLAB Function  TreatAsAtomicUnit=on
  Mixer : MATLAB Function  TreatAsAtomicUnit=on
  MotorsAndPropellers : MATLAB Function  TreatAsAtomicUnit=on
  Position : Integrator
  RotationalDynamics : MATLAB Function  TreatAsAtomicUnit=on
  RotationalVelocity : Integrator
  Velocity : Integrator
  acc_rpy : Outport
  vel_rpy : Outport  Port=2
  euler_rpy : Outport  Port=3
  acc_xyz : Outport  Port=4
  vel_xyz : Outport  Port=5
  pos_xyz : Outport  Port=6
  MotorCurrent : Outport  Port=7
  wires:
  MotorsAndPropellers/1(Torque) -> RotationalDynamics/1(Torque)
  RotationalDynamics/1(RotAcceleration) -> acc_rpy/1, RotationalVelocity/1
  RotationalVelocity/1 -> vel_rpy/1, RotationalDynamics/3(Omega), Angle/1
  MotorsAndPropellers/2(F) -> LinearDynamics/1(F), RotationalDynamics/2(F)
  Disturbance/1(DragDisturbance) -> LinearDynamics/2(Disturbance)
  Velocity/1 -> vel_xyz/1, LinearDynamics/4(Velocity), Position/1
  LinearDynamics/1(Acceleration) -> acc_xyz/1, Velocity/1
  Position/1 -> pos_xyz/1
  Roll/1 -> Mixer/3(Roll)
  WindDisturbance/1 -> Disturbance/1(VelocityDisturbance)
  Pitch/1 -> Mixer/2(Pitch)
  Mixer/1(Voltage) -> MotorsAndPropellers/1(Voltage)
  MotorsAndPropellers/3(Current) -> MotorCurrent/1
  Yaw/1 -> Mixer/4(Yaw)
  Angle/1 -> euler_rpy/1, LinearDynamics/3(Theta)
  Throttle/1 -> Mixer/1(Throttle)

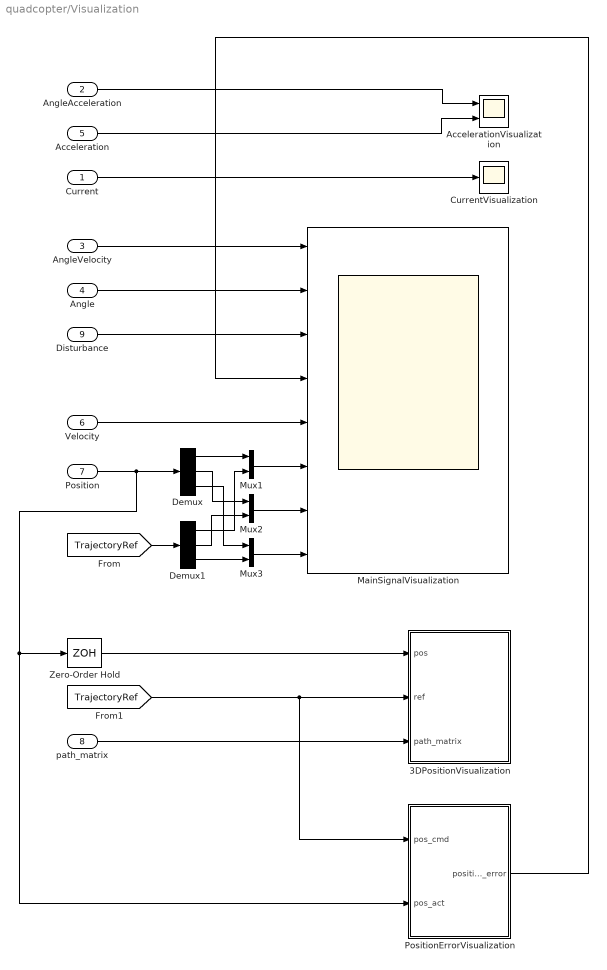
== system quadcopter/Visualization ==
  Current : Inport
  AngleAcceleration : Inport  Port=2
  AngleVelocity : Inport  Port=3
  Angle : Inport  Port=4
  Acceleration : Inport  Port=5
  Velocity : Inport  Port=6
  Position : Inport  Port=7
  path_matrix : Inport  Port=8
  Disturbance : Inport  Port=9
  3DPositionVisualization : MATLAB Function  TreatAsAtomicUnit=on
  AccelerationVisualization : Scope  NumInputPorts=2
  CurrentVisualization : Scope
  Demux : Demux  Outputs=3
  Demux1 : Demux  Outputs=3
  MainSignalVisualization : Scope  NumInputPorts=8
  Mux1 : Mux  Inputs=2
  Mux2 : Mux  Inputs=2
  Mux3 : Mux  Inputs=2
  PositionErrorVisualization : MATLAB Function  TreatAsAtomicUnit=on
  Zero-Order Hold : ZeroOrderHold  SampleTime=0.001
  wires:
  Demux1/1 -> Mux1/2
  Zero-Order Hold/1 -> 3DPositionVisualization/1(pos)
  Velocity/1 -> MainSignalVisualization/5
  path_matrix/1 -> 3DPositionVisualization/3(path_matrix)
  Mux3/1 -> MainSignalVisualization/8
  Demux/1 -> Mux1/1
  Mux1/1 -> MainSignalVisualization/6
  Mux2/1 -> MainSignalVisualization/7
  Demux1/2 -> Mux2/2
  Demux/2 -> Mux2/1
  Demux/3 -> Mux3/1
  [TrajectoryRef] -> 3DPositionVisualization/2(ref), PositionErrorVisualization/1(pos_cmd)
  [TrajectoryRef] -> Demux1/1
  Demux1/3 -> Mux3/2
  Current/1 -> CurrentVisualization/1
  Angle/1 -> MainSignalVisualization/2
  AngleVelocity/1 -> MainSignalVisualization/1
  Position/1 -> Demux/1, Zero-Order Hold/1, PositionErrorVisualization/2(pos_act)
  PositionErrorVisualization/1(position_error) -> MainSignalVisualization/4
  Disturbance/1 -> MainSignalVisualization/3
  AngleAcceleration/1 -> AccelerationVisualization/1
  Acceleration/1 -> AccelerationVisualization/2

== matlab function quadcopter/Guidance/TrajectoryPlanner ==
  settings: updateMethod=DISCRETE  sampleTime=0.05
  data: path_matrix output; traj_mode input
function path_matrix = fcn(traj_mode)
    % MASTER TRAJECTORY PLANNER
    % traj_mode: 1 = Helix, 2 = Figure-8
    
    % Strictly enforce the matrix size right at the start to protect the compiler
    path_matrix = zeros(200, 3);
    path_matrix(1, :) = [0, 0, 0];
    
    if traj_mode == 1
        % --- HELIX GENERATION ---
        path_matrix(2, :) = [0, 0, 2]; % Takeoff
        for i = 3:200
            t = (i - 3) * 0.5;
            path_matrix(i, 1) = 10 * sin(0.2 * t);
            path_matrix(i, 2) = 10 - 10 * cos(0.2 * t);
            path_matrix(i, 3) = 2 + (0.1 * t);
        end
        
    else
        % --- FIGURE-8 GENERATION ---
        path_matrix(2, :) = [0, 0, 5]; % Takeoff
        for i = 3:200
            t = (i - 3) * 0.5;
            path_matrix(i, 1) = 10 * sin(0.2 * t);
            path_matrix(i, 2) = 10 * sin(0.4 * t); % 2x frequency
            path_matrix(i, 3) = 5;
        end
    end
end

== matlab function quadcopter/Quadcopter/RotationalDynamics ==
  data: Torque input; RotAcceleration output size=[3,1]; F input; Omega input
function RotAcceleration = fcn(Torque, F, Omega)
side_length = 0.237; % m

p = Omega(1);
q = Omega(2);
r = Omega(3);

moment = zeros(3,1); % x y z
I = [0.003;
     0.003;
     0.007]; % kg.m2 - inertia

moment(1) = (F(3)+F(4))*side_length/2 - (F(1)+F(2))*side_length/2 ...
                                      + q*r*(I(2)-I(3));
moment(2) = (F(3)+F(2))*side_length/2 - (F(1)+F(4))*side_length/2 ...
                                      + p*r*(I(3)-I(1));
moment(3) = Torque(4) - Torque(1) + Torque(2) - Torque(3) ...
                                      + p*q*(I(1)-I(2));

RotAcceleration = moment ./I;

== matlab function quadcopter/Quadcopter/MotorsAndPropellers ==
  data: Voltage input; Torque output; F output; Current output
function [Torque, F, Current] = fcn(Voltage)
Kv  = 1400;   % RPM/V   - motor velocity constant
rho = 1.225;  % kg/m3   - air density 
D   = 0.2;    % m       - diameter of propeller

rpm     = [0 0 0 0];
Torque  = [0 0 0 0];
Current = [0 0 0 0];
F       = [0 0 0 0];

for i = 1:4
    rpm(i) = -2.6931*Voltage(i)^3 + Kv*Voltage(i);
    n = rpm(i)/60; % round per second
    Ct = 2*10^-15*rpm(i)^3 - 4*10^-11*rpm(i)^2 + 3*10^-7*rpm(i) + 0.1013;
    F(i) = Ct*rho*n^2*D^4;
    Torque(i) = 4*10^-14*rpm(i)^3 + 8*10^-12*rpm(i)^2 + 3*10^-6*rpm(i);
    Current(i) = Kv*Torque(i);
end

== matlab function quadcopter/Quadcopter/LinearDynamics ==
  data: F input; Disturbance input; Acceleration output; Theta input; Velocity input
function Acceleration = fcn(F, Disturbance, Theta, Velocity)
m = 0.743;
g = 9.81;
A = [0.0197 0.0197 0.0512]; % m2
rho = 1.225; % kg/m3 - air density
Cd = 1; % drag coef

Drag = [0 0 0];
for i = 1:3
    Drag(i) = 0.5*rho*Velocity(i)^2*A(i)*Cd;
end

Acceleration = [0 0 0];
Force = [0 0 0];
Fprop = [0 0 0];

Fprop(1) = sin(Theta(2))*cos(Theta(1))*(F(1)+F(2)+F(3)+F(4));
Fprop(2) = sin(Theta(1))*cos(Theta(2))*(F(1)+F(2)+F(3)+F(4));
Fprop(3) = cos(Theta(1))*cos(Theta(2))*(F(1)+F(2)+F(3)+F(4));

ThetaXY = -atan2(Fprop(1), Fprop(2));
XY2D = sqrt(Fprop(1)^2 + Fprop(2)^2);

if Fprop(3) >= 0
    Fprop(1) = XY2D*sin(ThetaXY+Theta(3));
    Fprop(2) = XY2D*cos(ThetaXY+Theta(3));
else
    Fprop(1) = XY2D*sin(ThetaXY-Theta(3));
    Fprop(2) = XY2D*cos(ThetaXY-Theta(3));
end

if Velocity(1) < 0
    Force(1) = Fprop(1) - Disturbance(1) + Drag(1);
else
    Force(1) = Fprop(1) - Disturbance(1) - Drag(1);
end

if Velocity(2) < 0
    Force(2) = Fprop(2) - Disturbance(2) + Drag(2);
else
    Force(2) = Fprop(2) - Disturbance(2) - Drag(2);
end

if Velocity(3) < 0
    Force(3) = Fprop(3) - Disturbance(3) + Drag(3) - m*g;
else
    Force(3) = Fprop(3) - Disturbance(3) - Drag(3) - m*g;
end

for i = 1:3
    Acceleration(i) = Force(i)/m;
end

== matlab function quadcopter/Quadcopter/Disturbance ==
  data: VelocityDisturbance input; DragDisturbance output
function DragDisturbance = fcn(VelocityDisturbance)
A = [0.0197 0.0197 0.0197*2*1.3];
DragDisturbance = [0 0 0];
rho = 1.225;
Cd = 1;

for i = 1:3
    if VelocityDisturbance(i) < 0
        DragDisturbance(i) = 0.5*rho*VelocityDisturbance(i)^2*A(i)*Cd;
    else
        DragDisturbance(i) = -0.5*rho*VelocityDisturbance(i)^2*A(i)*Cd;
    end
end

== matlab function quadcopter/Quadcopter/Mixer ==
  data: Throttle input; Voltage output; Pitch input; Roll input; Yaw input
function Voltage = fcn(Throttle, Pitch, Roll, Yaw)
    % 1. Create local variables to avoid modifying read-only inputs
    p = Pitch;
    r = Roll;
    y = Yaw;
    Correct = 0;
    
    % 2. Calculate corrections
    if (p/2 + r/2 + y/2) > (100 - Throttle)
        Correct = (p/2 + r/2 + y/2) - (100 - Throttle);
    end
    if (p/2 + r/2 + y/2) > Throttle   % make sure the power never shut off
        if Correct < ((p/2 + r/2 + y/2) - Throttle)
            Correct = (p/2 + r/2 + y/2) - Throttle;
        end
    end
    
    if Correct ~= 0
        p = p - Correct/3*2;
        r = r - Correct/3*2;
        y = y - Correct/3*2;
    end
    
    % 3. PREALLOCATE the Voltage array to satisfy the Simulink Coder
    Voltage = zeros(4,1);
    
    % 4. Assign the voltages using the local variables
    Voltage(1) = (Throttle - p/2 - r/2 - y/2) * 11.4 / 100;     % altitude
    Voltage(2) = (Throttle - p/2 + r/2 + y/2) * 11.4 / 100;     % forward/backward
    Voltage(3) = (Throttle + p/2 + r/2 - y/2) * 11.4 / 100;     % right/left
    Voltage(4) = (Throttle + p/2 - r/2 + y/2) * 11.4 / 100;     % yaw
    
    % 5. Prevent negative voltage physics errors
    for i = 1:4
        if Voltage(i) < 0
            Voltage(i) = 0;
        elseif Voltage(i) > 11.4
            Voltage(i) = 11.4;
        end
    end
end

== matlab function quadcopter/Visualization/3DPositionVisualization ==
  settings: updateMethod=DISCRETE  sampleTime=0.005
  data: pos input; ref input; path_matrix input
function visualize_position(pos, ref, path_matrix)
    coder.extrinsic('plot3', 'drawnow', 'figure', 'set', 'grid', 'xlabel', 'ylabel', 'zlabel', 'legend', 'hold', 'axis', 'view');
    
    persistent fig hArms hProps hTrail hTarget hRefLine trailX trailY trailZ stepCount render_skip
    
    if isempty(stepCount)
        stepCount = 1;
        render_skip = 0; % Initialize frame decimation counter
        trailX = nan(1, 100000); trailY = nan(1, 100000); trailZ = nan(1, 100000);
    end
    
    % INITIALIZATION PHASE
    if isempty(fig)
        fig = 1; 
        figure('Name', 'Live 3D Flight Path'); hold('on');
        
        hRefLine = plot3(path_matrix(:,1), path_matrix(:,2), path_matrix(:,3), 'r--', 'LineWidth', 1.5);
        hTrail = plot3(trailX, trailY, trailZ, 'b-', 'LineWidth', 1.5);
        hTarget = plot3(nan, nan, nan, 'ro', 'MarkerFaceColor', 'r', 'MarkerSize', 6);
        
        hArms = plot3(nan(1,5), nan(1,5), nan(1,5), 'k-', 'LineWidth', 2); 
        hProps = plot3(nan(1,4), nan(1,4), nan(1,4), 'bo', 'MarkerFaceColor', 'b', 'MarkerSize', 6); 
        
        grid('on'); xlabel('X (m)'); ylabel('Y (m)'); zlabel('Altitude (m)');
        legend('Reference Path', 'Real Trajectory', 'Current Target', 'Location', 'best');
        axis([-15 25 -15 25 0 30]); view(45, 30); 
    end
    
    % REAL-TIME LOGGING (Runs every step so the blue line is perfectly accurate)
    pos = pos(:); ref = ref(:);
    if stepCount <= 100000
        trailX(stepCount) = pos(1); trailY(stepCount) = pos(2); trailZ(stepCount) = pos(3);
        stepCount = stepCount + 1;
    end
    
    % FRAME DECIMATION: Only redraw the 3D plot every 20 steps
    render_skip = render_skip + 1;
    
    if render_skip >= 20
        set(hTrail, 'XData', trailX, 'YData', trailY, 'ZData', trailZ);
        set(hRefLine, 'XData', path_matrix(:,1), 'YData', path_matrix(:,2), 'ZData', path_matrix(:,3));
        set(hTarget, 'XData', ref(1), 'YData', ref(2), 'ZData', ref(3));
        
        L = 1.0; 
        p1 = [L; 0; 0] + pos; p2 = [-L; 0; 0] + pos; p3 = [0; L; 0] + pos; p4 = [0; -L; 0] + pos;
        armX = [p1(1), p2(1), NaN, p3(1), p4(1)]; armY = [p1(2), p2(2), NaN, p3(2), p4(2)]; armZ = [p1(3), p2(3), NaN, p3(3), p4(3)];
        propX = [p1(1), p2(1), p3(1), p4(1)]; propY = [p1(2), p2(2), p3(2), p4(2)]; propZ = [p1(3), p2(3), p3(3), p4(3)];
        
        set(hArms, 'XData', armX, 'YData', armY, 'ZData', armZ); set(hProps, 'XData', propX, 'YData', propY, 'ZData', propZ);
        
        drawnow limitrate;
        render_skip = 0; % Reset counter
    end
end

== matlab function quadcopter/Controller/WorldToBody Kinematics ==
  data: Ux input; DesiredPitch output; Uy input; Yaw input; DesiredRoll output
function [DesiredPitch, DesiredRoll] = fcn(Ux, Uy, Yaw)
    % Ux is the control effort from the X-Axis PID
    % Uy is the control effort from the Y-Axis PID
    % Yaw is the current heading feedback (from euler_rpy)
    
    % transform world-frame translational into body-frame tilt angles
    DesiredRoll  = -Ux * cos(Yaw) + Uy * sin(Yaw);
    DesiredPitch =  Ux * sin(Yaw) + Uy * cos(Yaw);
end

== matlab function quadcopter/TrajectoryGenerator ==
  data: t input; X_cmd output; Y_cmd output; Z_cmd output
function [X_cmd, Y_cmd, Z_cmd] = fcn(t)
    % SLOWER GUIDANCE NODE: Generates a 3D Helix Trajectory over 100s
    
    radius = 10;       
    omega = 0.2;       % Reduced from 0.5 to make it fly much slower
    climb_rate = 0.2;  % Reduced from 0.5 for a gentle ascent
    
    if t < 5
        % Hover for 5 seconds to stabilize
        X_cmd = 0;
        Y_cmd = 0;
        Z_cmd = 2; 
    else
        % Begin slower, 95-second spiral trajectory
        time = t - 5; 
        X_cmd = radius * sin(omega * time);
        Y_cmd = radius * cos(omega * time);
        Z_cmd = 2 + (climb_rate * time);
    end
end
